simulink model "Motor_and_Driver"  (R2020a)
settings: Solver=VariableStepAuto  StartTime=0.0  StopTime=10.0  RelTol=1e-3
model workspace (MAT data in the model file):
  C = [700; 0.9999]
  K = 70.3
  KdPEPOS4 = 1
  KiIEPOS4 = 1
  KiPEPOS4 = 1
  KpIPEPOS4 = 1
  KpPEPOS4 = 1
  Ts = 0.02
  g = 0.1507
  m = 90.5176213536
  q = 0.1507
  tau = 0.0127
undefined symbols (not defined in the file): A, Angle, B, Current, DiscIntNeverNeededParam, f_DIncrEnc, Speed, Torque
libraries: fl_lib x24, nesl_utility x15, ee_lib x7, simulink x4, powerlib_meascontrol x1
settings Model: DataDictionary=MotorInfo.sldd  OrderedModelArguments=off  Creator=khoi  LastModifiedBy=khoi
settings SolverCC: AlgebraicLoopSolver=LineSearch
settings DataIOCC: SaveFormat=Structure  SaveOutput=off
settings DebuggingCC: AlgebraicLoopMsg=none
settings ModelReferenceCC: EnableParallelModelReferenceBuilds=on
settings RTWCC: GenCodeOnly=on

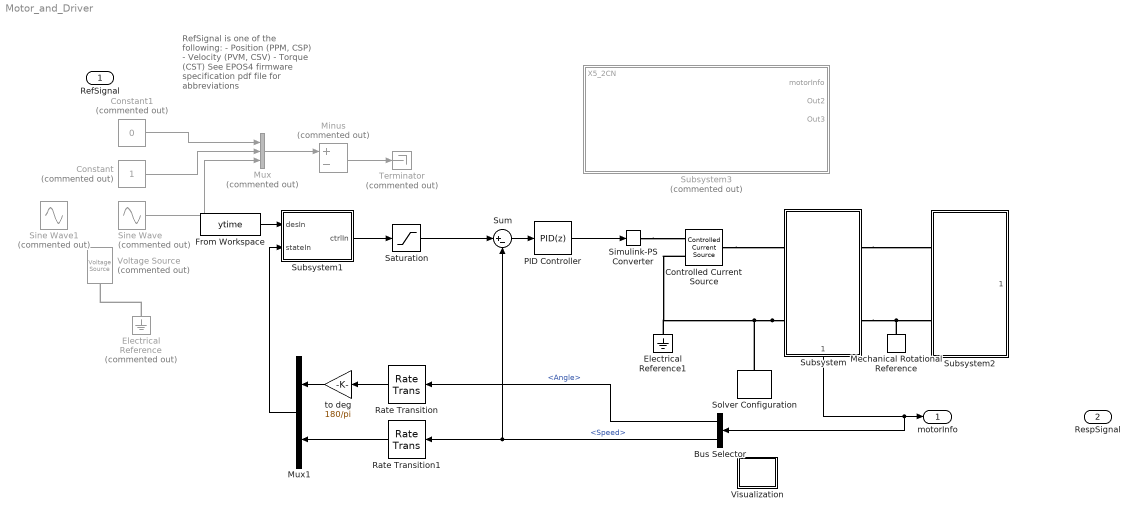
== system Motor_and_Driver ==
  note: RefSignal is one of the following:
      | - Position (PPM, CSP)
      | - Velocity (PVM, CSV)
      | - Torque (CST)
      | See EPOS4 firmware specification pdf file for abbreviations
  RefSignal : Inport
  Bus Selector : BusSelector  OutputSignals=Angle,Speed
  Constant : Constant  Commented=on
  Constant1 : Constant  Commented=on  Value=0
  Controlled Current Source : fl_lib/Electrical/Electrical Sources/Controlled Current Source
  Electrical Reference : fl_lib/Electrical/Electrical Elements/Electrical Reference  Commented=on
      settings: SourceProductBaseCode=MT,SS
  Electrical Reference1 : fl_lib/Electrical/Electrical Elements/Electrical Reference
      settings: SourceProductBaseCode=MT,SS
  From Workspace : FromWorkspace  VariableName=ytime  SampleTime=Ts  OutputAfterFinalValue=Holding final value
  Mechanical Rotational Reference : fl_lib/Mechanical/Rotational Elements/Mechanical Rotational Reference
  Minus : Sum  Commented=on  Inputs=+-
  Mux : Mux  Commented=on  Inputs=3
  Mux1 : Mux  Inputs=2
  PID Controller : simulink/Continuous/PID Controller  Controller=PID  Form=Parallel  TimeDomain=Discrete-time  UseExternalTs=off  SampleTime=Ts  IntegratorMethod=Forward Euler  FilterMethod=Forward Euler  ControllerParametersSource=internal  P=-3.52033117976818  I=-1.96454147896898  D=-0.000784751618376711  UseFilter=on  N=70.0522807561808  TunerSelectOption=Transfer Function Based (PID Tuner App)  InitialConditionSource=internal  InitialConditionForIntegrator=0  InitialConditionForFilter=0  DifferentiatorICPrevScaledInput=0  ExternalReset=none  TrackingMode=off  Kt=1  LimitOutput=on  UpperSaturationLimit=15  LowerSaturationLimit=-15  LinearizeAsGain=on  AntiWindupMode=none  Kb=1  POutMin=[]  POutMax=[]  IOutMin=[]  IOutMax=[]  DOutMin=[]  DOutMax=[]  NOutMin=[]  NOutMax=[]  SumOutMin=[]  SumOutMax=[]  SaturationOutMin=[]  SaturationOutMax=[]  PParamMin=[]  PParamMax=[]  IParamMin=[]  IParamMax=[]  DParamMin=[]  DParamMax=[]  NParamMin=[]  NParamMax=[]  KbParamMin=[]  KbParamMax=[]  KtParamMin=[]  KtParamMax=[]  KbOutMin=[]  KbOutMax=[]  KtOutMin=[]  KtOutMax=[]  IntegratorOutMin=[]  IntegratorOutMax=[]  FilterOutMin=[]  FilterOutMax=[]  SumI1OutMin=[]  SumI1OutMax=[]  SumI2OutMin=[]  SumI2OutMax=[]  SumI3OutMin=[]  SumI3OutMax=[]  SumI4OutMin=[]  SumI4OutMax=[]  SumDOutMin=[]  SumDOutMax=[]  DifferentiatorOutMin=[]  DifferentiatorOutMax=[]  FilterDiffOutCoefMin=[]  FilterDiffOutCoefMax=[]  ReciprocalOutMin=[]  ReciprocalOutMax=[]  SumDenOutMin=[]  SumDenOutMax=[]  SumNumOutMin=[]  SumNumOutMax=[]  DivideOutMin=[]  DivideOutMax=[]  UdiffTsProdOutMin=[]  UdiffTsProdOutMax=[]  NTsProdOutMin=[]  NTsProdOutMax=[]  UintegralTsProdOutMin=[]  UintegralTsProdOutMax=[]  UngainTsProdOutMin=[]  UngainTsProdOutMax=[]  IntegratorContinuousStateAttributes=''  IntegratorStateMustResolveToSignalObject=off  IntegratorRTWStateStorageClass=Auto  FilterContinuousStateAttributes=''  FilterStateMustResolveToSignalObject=off  FilterRTWStateStorageClass=Auto  ParallelPVariant=InternalParameters  IdealPVariant=Disabled  IVariant=InternalParameters  DVariant=InternalParameters  IntegratorVariant=Discrete  SatVariant=Enabled  AWVariant=Passthrough  PCopyVariant=Disabled  TRVariant=Disabled  FdbkBlocksVariant=Forward  IdealPFdbkVariant=Disabled  SatFdbkVariant=Disabled  DerivativeFilterVariant=ForwardEulerFilter  NVariant=InternalParameters  NCopyVariant=Disabled  FilterICVariant=InternalICsFilter  IntegratorICVariant=InternalICs  ExternalResetVariant=Disabled  TRSumVariant=Passthrough  SumFdbkVariant=Disabled  SumVariant=Sum_PID  TsampFilterVariant=InternalTs  TsampNgainVariant=Passthrough  TsampIntegralVariant=Passthrough
  Rate Transition : RateTransition  OutPortSampleTime=Ts
  Rate Transition1 : RateTransition  OutPortSampleTime=Ts
  Saturation : Saturate  UpperLimit=2100  LowerLimit=-2100
  Simulink-PS Converter : nesl_utility/Simulink-PS Converter  PhysicalDomain=network_engine_domain  SubClassName=ps_input  LeftPortType=input  RightPortType=output  PseudoPeriodic=off  Frequencies=[]  NoiseDistribution=none  NoiseParameters=[]  Unit=1  AffineConversion=off  FilteringAndDerivatives=provide  SimscapeFilterOrder=1  InputFilterTimeConstant=0.001  UdotUserProvided=0
  Sine Wave : Sin  Commented=on  Amplitude=5  SampleTime=0
  Sine Wave1 : Sin  Commented=on  Amplitude=400  Bias=0.5  SampleTime=Ts
  Solver Configuration : nesl_utility/Solver Configuration  PhysicalDomain=network_engine_domain  SubClassName=solver  LeftPortType=input  RightPortType=generic  Tones=[]  Harmonics=[]  SimulateNoise=off  Profile=off  UseLocalSampling=off  EnableSwitchedLinearOptims=on  FrequencyDomain=off  UseCCode=off  RelTol=0.001  AbsTol=1e-06  MinStep=1e-09  ToWorkspace=off  RevertToSquareIcSolve=off  NumHomotopyIterations=100  PhasorMode=off  PhasorModeNumHarmonics=1  DoDC=off  ResidualTolerance=1e-09  UseLocalSolver=off  LocalSolverChoice=NE_BACKWARD_EULER_ADVANCER  LocalSolverSampleTime=0.001  DoFixedCost=off  MaxNonlinIter=3  MaxModeIter=2  LinearAlgebra=auto  EquationFormulation=NE_TIME_EF  DelaysMemoryBudget=1024  AutomaticFiltering=on  FilteringTimeConstant=0.001  PartitionStorageMethod=AS_NEEDED  PartitionMemoryBudget=1024  PartitionMethod=ROBUST
  Subsystem : Subsystem  ReferencedSubsystem=Motor
      settings: PortSchema="{\"entries\":[{\"content\":{\"sides\":[{\"content\":{\"connectorIds\":[\"LConn2\",\"LConn1\"]},\"type\":\"ConnectorPlacement.EquallySpacedRectSide\",\"uuid\":\"2c9fa8b8-125e-4798-9362-86aeecc8fa1f\"},{\"content\":{\"connectorIds\":[\"LConn3\",\"LConn4\"],\"side\":\"RIGHT\"},\"type\":\"ConnectorPlacement.EquallySpacedRectSide\",\"uuid\":\"4f69e704-bc05-469f-ab35-d6b84ad80397\"},{\"content\":{\"connectorIds\":[],\"side\":\"TOP\"},\"type\":\"ConnectorPlacement.EquallySpacedRectSide\",\"uuid\":\"cfaf3aee-cd20-40cb-9288-e8b7cf9f1276\"},{\"content\":{\"connectorIds\":[\"Out1\"],\"side\":\"BOTTOM\"},\"type\":\"ConnectorPlacement.EquallySpacedRectSide\",\"uuid\":\"777429de-77ae-4f2a-b3d7-49600205512c\"}]},\"type\":\"ConnectorPlacement.EquallySpacedConnector\",\"uuid\":\"9e55bc0d-63a8-4cde-b859-9b2193dba80d\"}],\"packageUris\":[\"http://schema.mathworks.com/mf0/Connector/19700101\"],\"version\":\"1.0\"}"
  Subsystem1 : Subsystem
  Subsystem2 : Subsystem  ReferencedSubsystem=Loads
  Subsystem3 : Subsystem  Commented=on
  Sum : Sum  Inputs=|+-
  Terminator : Terminator  Commented=on
  Visualization : Subsystem
  Voltage Source : ee_lib/Sources/Voltage Source  Commented=on  dc_voltage=x607325_VNom V  ac_voltage=0 V  ac_shift=0 rad  ac_frequency=60 Hz  noise_mode=0  PSD=0 V^2/Hz  repeatability=1  auto_seed=396848355  user_seed=0  sample_time=1e-3 s  i_specify=off  i_priority=None  i=0 A  i_nominal_specify=off  i_nominal_unit=A  i_nominal_value=1  v_specify=off  v_priority=None  v=0 V  v_nominal_specify=off  v_nominal_unit=V  v_nominal_value=1
  to deg : Gain  Gain=180/pi
  motorInfo : Outport  OutDataTypeStr=Bus: motorInfo
  RespSignal : Outport  Port=2  OutDataTypeStr=Bus: RespSignal
  wires:
  Mux/1 -> Minus/1
  Subsystem/1 -> Bus Selector/1, motorInfo/1
  Minus/1 -> Terminator/1
  ? -> RespSignal/1
  Sine Wave/1 -> Mux/3
  Constant/1 -> Mux/2
  Constant1/1 -> Mux/1
  Saturation/1 -> Sum/1
  PID Controller/1 -> Simulink-PS Converter/1
  Bus Selector/2 -> Sum/2, Rate Transition1/1  "<Speed>"
  Sum/1 -> PID Controller/1
  From Workspace/1 -> Subsystem1/1(desIn)
  Subsystem1/1(ctrlIn) -> Saturation/1
  Bus Selector/1 -> Rate Transition/1  "<Angle>"
  Rate Transition/1 -> to deg/1
  to deg/1 -> Mux1/1
  Rate Transition1/1 -> Mux1/2
  Mux1/1 -> Subsystem1/2(stateIn)
  connections:
  Subsystem/LConn1 -- Solver Configuration/RConn1 -- Controlled Current Source/RConn2 -- Electrical Reference1/LConn1
  Controlled Current Source/LConn1 -- Subsystem/LConn2
  Electrical Reference/LConn1 -- Voltage Source/RConn1
  Simulink-PS Converter/RConn1 -- Controlled Current Source/RConn1
  Mechanical Rotational Reference/LConn1 -- Subsystem2/LConn2 -- Subsystem/LConn4
  Subsystem/LConn3 -- Subsystem2/LConn1

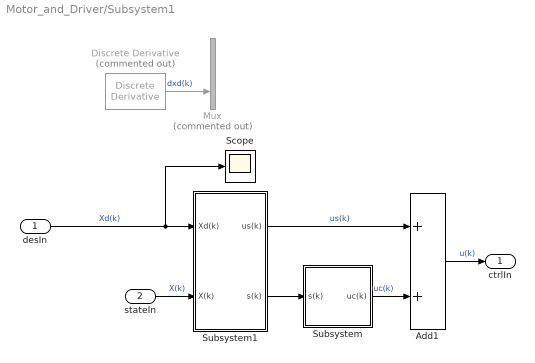
== system Motor_and_Driver/Subsystem1 ==
  desIn : Inport
  stateIn : Inport  Port=2  PortDimensions=2
  Add1 : Sum
  Discrete Derivative : simulink/Discrete/Discrete Derivative  Commented=on  gainval=1.0  ICPrevScaledInput=0.0  OutMin=[]  OutMax=[]  OutDataType=fixdt(1, 16)  OutScaling=2^-10  DoSatur=off
  Mux : Mux  Commented=on  Inputs=2
  Scope : Scope
  Subsystem : Subsystem
  Subsystem1 : Subsystem
  ctrlIn : Outport
  wires:
  desIn/1 -> Scope/1, Subsystem1/1(Xd(k))  "Xd(k)"
  Subsystem1/1(us(k)) -> Add1/1  "us(k)"
  stateIn/1 -> Subsystem1/2(X(k))  "X(k)"
  Subsystem/1(uc(k)) -> Add1/2  "uc(k)"
  Subsystem1/2(s(k)) -> Subsystem/1(s(k))
  Add1/1 -> ctrlIn/1  "u(k)"
  Discrete Derivative/1 -> Mux/2  "dxd(k)"

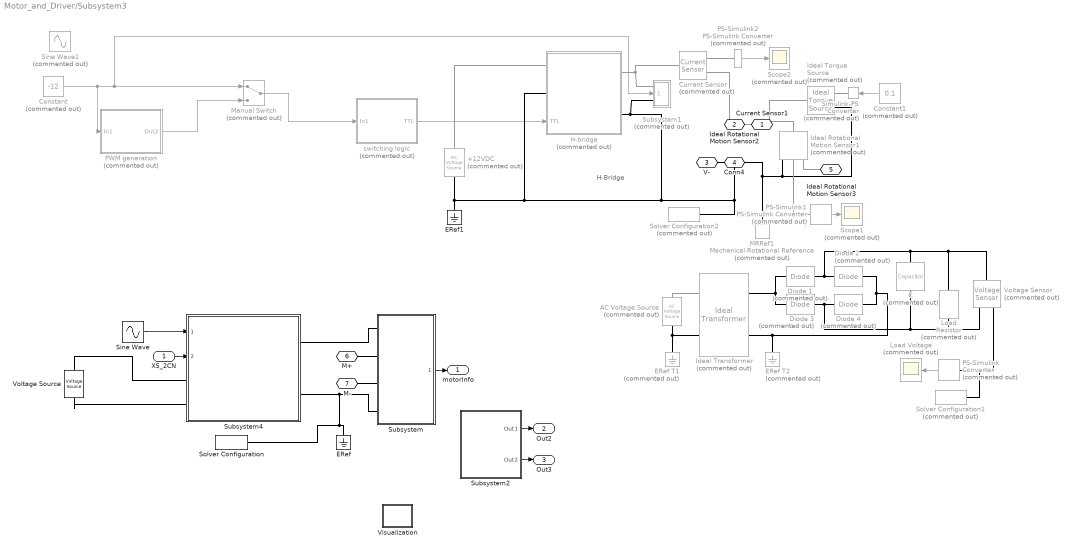
== system Motor_and_Driver/Subsystem3 ==
  note: H-Bridge
  X5_2CN : Inport
  +12VDC : fl_lib/Electrical/Electrical Sources/DC Voltage Source  Commented=on  v0=12 V
      settings: SourceProductBaseCode=MT,SS
  AC Voltage Source : fl_lib/Electrical/Electrical Sources/AC Voltage Source  Commented=on  amp=sqrt(2)*120 V  shift=0 deg  frequency=60 Hz  omega=0 rad/s
      settings: SourceProductBaseCode=MT,SS
  C : fl_lib/Electrical/Electrical Elements/Capacitor  Commented=on  c=470e-06 F  r=1e-06 Ohm  g=0 1/Ohm  i_specify=off  i_priority=High  i=0 A  i_nominal_specify=off  i_nominal_unit=A  i_nominal_value=1  v_specify=off  v_priority=High  v=0 V  v_nominal_specify=off  v_nominal_unit=V  v_nominal_value=1  vc_specify=on  vc_priority=High  vc=0 V  vc_nominal_specify=off  vc_nominal_unit=V  vc_nominal_value=1
      settings: SourceProductBaseCode=MT,SS
  Constant : Constant  Commented=on  Value=-12
  Constant1 : Constant  Commented=on  Value=0.1
  Current Sensor : fl_lib/Electrical/Electrical Sensors/Current Sensor  Commented=on
  Diode {1..4} (4 alike) : fl_lib/Electrical/Electrical Elements/Diode  Commented=on  Vf=0.6 V  Ron=0.3 Ohm  Goff=1e-08 1/Ohm  i_specify=off  i_priority=High  i=0 A  i_nominal_specify=off  i_nominal_unit=A  i_nominal_value=1  v_specify=off  v_priority=High  v=0 V  v_nominal_specify=off  v_nominal_unit=V  v_nominal_value=1
      settings: SourceProductBaseCode=MT,SS
  ERef : fl_lib/Electrical/Electrical Elements/Electrical Reference
      settings: SourceProductBaseCode=MT,SS
  ERef T1 : fl_lib/Electrical/Electrical Elements/Electrical Reference  Commented=on
      settings: SourceProductBaseCode=MT,SS
  ERef T2 : fl_lib/Electrical/Electrical Elements/Electrical Reference  Commented=on
      settings: SourceProductBaseCode=MT,SS
  ERef1 : fl_lib/Electrical/Electrical Elements/Electrical Reference
      settings: SourceProductBaseCode=MT,SS
  H-bridge : Subsystem  Commented=on
      settings: PortSchema="{\"entries\":[{\"content\":{\"sides\":[{\"content\":{\"connectorIds\":[\"LConn1\",\"LConn2\",\"In1\"]},\"type\":\"ConnectorPlacement.EquallySpacedRectSide\",\"uuid\":\"fc5f9395-6fe0-4e46-ba71-86f87805e004\"},{\"content\":{\"connectorIds\":[\"RConn1\",\"RConn2\"],\"side\":\"RIGHT\"},\"type\":\"ConnectorPlacement.EquallySpacedRectSide\",\"uuid\":\"2ca15bd9-a54f-419c-a915-39989ac75dc3\"},{\"content\":{\"connectorIds\":[],\"side\":\"TOP\"},\"type\":\"ConnectorPlacement.EquallySpacedRectSide\",\"uuid\":\"650dbc47-32e7-4b39-ba0c-96beec205e1a\"}]},\"type\":\"ConnectorPlacement.EquallySpacedConnector\",\"uuid\":\"775f97cb-687e-4894-86d4-689d0d470dfc\"}],\"packageUris\":[\"http://schema.mathworks.com/mf0/Connector/19700101\"],\"version\":\"1.0\"}"
  Ideal Rotational Motion Sensor1 : fl_lib/Mechanical/Mechanical Sensors/Ideal Rotational Motion Sensor  Commented=on  wrap_angle=simscape.enum.onoff.off  offset=0 deg
      settings: SourceProductBaseCode=MT,SS
  Ideal Torque Source : fl_lib/Mechanical/Mechanical Sources/Ideal Torque Source  Commented=on
  Ideal Transformer : fl_lib/Electrical/Electrical Elements/Ideal Transformer  Commented=on  n=14  i1_specify=off  i1_priority=High  i1=0 A  i1_nominal_specify=off  i1_nominal_unit=A  i1_nominal_value=1  v1_specify=off  v1_priority=High  v1=0 V  v1_nominal_specify=off  v1_nominal_unit=V  v1_nominal_value=1  i2_specify=off  i2_priority=High  i2=0 A  i2_nominal_specify=off  i2_nominal_unit=A  i2_nominal_value=1  v2_specify=off  v2_priority=High  v2=0 V  v2_nominal_specify=off  v2_nominal_unit=V  v2_nominal_value=1
      settings: SourceProductBaseCode=MT,SS
  Load : fl_lib/Electrical/Electrical Elements/Resistor  Commented=on  R=100 Ohm  i_specify=off  i_priority=High  i=0 A  i_nominal_specify=off  i_nominal_unit=A  i_nominal_value=1  v_specify=off  v_priority=High  v=0 V  v_nominal_specify=off  v_nominal_unit=V  v_nominal_value=1
      settings: SourceProductBaseCode=MT,SS
  Load Voltage : Scope  Commented=on
  MRRef1 : fl_lib/Mechanical/Rotational Elements/Mechanical Rotational Reference  Commented=on
      settings: SourceProductBaseCode=MT,SS
  Manual Switch : ManualSwitch  Commented=on
  PS-Simulink Converter : nesl_utility/PS-Simulink Converter  Commented=on  PhysicalDomain=network_engine_domain  SubClassName=ps_output  LeftPortType=input  RightPortType=output  PseudoPeriodic=off  Frequencies=[]  Unit=1  AffineConversion=off
      settings: SourceProductBaseCode=MT,SS
  PS-Simulink1 : nesl_utility/PS-Simulink Converter  Commented=on  PhysicalDomain=network_engine_domain  SubClassName=ps_output  LeftPortType=input  RightPortType=output  PseudoPeriodic=off  Frequencies=[]  Unit=rpm  AffineConversion=off
      settings: SourceProductBaseCode=MT,SS
  PS-Simulink2 : nesl_utility/PS-Simulink Converter  Commented=on  PhysicalDomain=network_engine_domain  SubClassName=ps_output  LeftPortType=input  RightPortType=output  PseudoPeriodic=off  Frequencies=[]  Unit=inherit  AffineConversion=off
      settings: SourceProductBaseCode=MT,SS
  PWM generation : Subsystem  Commented=on
  Scope1 : Scope  Commented=on
  Scope2 : Scope  Commented=on
  Simulink-PS Converter : nesl_utility/Simulink-PS Converter  Commented=on  PhysicalDomain=network_engine_domain  SubClassName=ps_input  LeftPortType=input  RightPortType=output  PseudoPeriodic=off  Frequencies=[]  NoiseDistribution=none  NoiseParameters=[]  Unit=1  AffineConversion=off  FilteringAndDerivatives=provide  SimscapeFilterOrder=1  InputFilterTimeConstant=0.001  UdotUserProvided=0
  Sine Wave : Sin  Amplitude=12  SampleTime=0
  Sine Wave1 : Sin  Commented=on  Amplitude=12  SampleTime=0.01
  Solver Configuration : nesl_utility/Solver Configuration  PhysicalDomain=network_engine_domain  SubClassName=solver  LeftPortType=input  RightPortType=generic  Tones=[]  Harmonics=[]  SimulateNoise=off  Profile=off  UseLocalSampling=off  EnableSwitchedLinearOptims=on  FrequencyDomain=off  UseCCode=off  RelTol=0.001  AbsTol=1e-06  MinStep=1e-09  ToWorkspace=off  RevertToSquareIcSolve=off  NumHomotopyIterations=100  PhasorMode=off  PhasorModeNumHarmonics=1  DoDC=off  ResidualTolerance=1e-9  UseLocalSolver=off  LocalSolverChoice=NE_BACKWARD_EULER_ADVANCER  LocalSolverSampleTime=5e-6  DoFixedCost=off  MaxNonlinIter=4  MaxModeIter=2  LinearAlgebra=auto  EquationFormulation=NE_TIME_EF  DelaysMemoryBudget=1024  AutomaticFiltering=on  FilteringTimeConstant=0.001  PartitionStorageMethod=AS_NEEDED  PartitionMemoryBudget=1024  PartitionMethod=FAST
      settings: SourceProductBaseCode=MT,SS
  Solver Configuration1 : nesl_utility/Solver Configuration  Commented=on  PhysicalDomain=network_engine_domain  SubClassName=solver  LeftPortType=input  RightPortType=generic  Tones=[]  Harmonics=[]  SimulateNoise=off  Profile=off  UseLocalSampling=off  EnableSwitchedLinearOptims=on  FrequencyDomain=off  UseCCode=off  RelTol=0.001  AbsTol=1e-06  MinStep=1e-09  ToWorkspace=off  RevertToSquareIcSolve=off  NumHomotopyIterations=100  PhasorMode=off  PhasorModeNumHarmonics=1  DoDC=off  ResidualTolerance=1e-9  UseLocalSolver=off  LocalSolverChoice=NE_BACKWARD_EULER_ADVANCER  LocalSolverSampleTime=.001  DoFixedCost=off  MaxNonlinIter=3  MaxModeIter=2  LinearAlgebra=auto  EquationFormulation=NE_TIME_EF  DelaysMemoryBudget=1024  AutomaticFiltering=on  FilteringTimeConstant=0.001  PartitionStorageMethod=AS_NEEDED  PartitionMemoryBudget=1024  PartitionMethod=FAST
      settings: SourceProductBaseCode=MT,SS
  Solver Configuration2 : nesl_utility/Solver Configuration  Commented=on  PhysicalDomain=network_engine_domain  SubClassName=solver  LeftPortType=input  RightPortType=generic  Tones=[]  Harmonics=[]  SimulateNoise=off  Profile=off  UseLocalSampling=off  EnableSwitchedLinearOptims=on  FrequencyDomain=off  UseCCode=off  RelTol=0.001  AbsTol=1e-06  MinStep=1e-09  ToWorkspace=off  RevertToSquareIcSolve=off  NumHomotopyIterations=100  PhasorMode=off  PhasorModeNumHarmonics=1  DoDC=off  ResidualTolerance=1e-9  UseLocalSolver=off  LocalSolverChoice=NE_BACKWARD_EULER_ADVANCER  LocalSolverSampleTime=5e-6  DoFixedCost=off  MaxNonlinIter=4  MaxModeIter=2  LinearAlgebra=auto  EquationFormulation=NE_TIME_EF  DelaysMemoryBudget=1024  AutomaticFiltering=on  FilteringTimeConstant=0.001  PartitionStorageMethod=AS_NEEDED  PartitionMemoryBudget=1024  PartitionMethod=FAST
      settings: SourceProductBaseCode=MT,SS
  Subsystem : Subsystem  ReferencedSubsystem=Motor
      settings: PortSchema="{\"entries\":[{\"content\":{\"sides\":[{\"content\":{\"connectorIds\":[\"LConn2\",\"LConn3\",\"LConn4\",\"LConn1\"]},\"type\":\"ConnectorPlacement.EquallySpacedRectSide\",\"uuid\":\"2c9fa8b8-125e-4798-9362-86aeecc8fa1f\"},{\"content\":{\"connectorIds\":[\"Out1\"],\"side\":\"RIGHT\"},\"type\":\"ConnectorPlacement.EquallySpacedRectSide\",\"uuid\":\"4f69e704-bc05-469f-ab35-d6b84ad80397\"},{\"content\":{\"connectorIds\":[],\"side\":\"TOP\"},\"type\":\"ConnectorPlacement.EquallySpacedRectSide\",\"uuid\":\"cfaf3aee-cd20-40cb-9288-e8b7cf9f1276\"}]},\"type\":\"ConnectorPlacement.EquallySpacedConnector\",\"uuid\":\"9e55bc0d-63a8-4cde-b859-9b2193dba80d\"}],\"packageUris\":[\"http://schema.mathworks.com/mf0/Connector/19700101\"],\"version\":\"1.0\"}"
  Subsystem1 : Subsystem  Commented=on
      settings: PortSchema="{\"entries\":[{\"content\":{\"sides\":[{\"content\":{\"connectorIds\":[]},\"type\":\"ConnectorPlacement.EquallySpacedRectSide\",\"uuid\":\"8985f9b9-7c8e-48a1-a039-7cc5a202e797\"},{\"content\":{\"connectorIds\":[\"RConn1\",\"In1\",\"RConn2\"],\"side\":\"RIGHT\"},\"type\":\"ConnectorPlacement.EquallySpacedRectSide\",\"uuid\":\"648da9d7-23ce-4076-bbaa-8fdefddefded\"},{\"content\":{\"connectorIds\":[],\"side\":\"TOP\"},\"type\":\"ConnectorPlacement.EquallySpacedRectSide\",\"uuid\":\"a83ba4c6-f8c4-4c80-b17f-0923e79ebda2\"}]},\"type\":\"ConnectorPlacement.EquallySpacedConnector\",\"uuid\":\"c20a9845-b952-47be-a6da-fffd20a0a984\"}],\"packageUris\":[\"http://schema.mathworks.com/mf0/Connector/19700101\"],\"version\":\"1.0\"}"
  Subsystem2 : Subsystem
  Subsystem4 : Subsystem  ReferencedSubsystem=EPOS4
      settings: PortSchema="{\"entries\":[{\"content\":{\"sides\":[{\"content\":{\"connectorIds\":[\"In1\",\"In2\",\"LConn3\",\"LConn4\"]},\"type\":\"ConnectorPlacement.EquallySpacedRectSide\",\"uuid\":\"8249666a-dc46-49ae-baa8-33cf79e5fc7b\"},{\"content\":{\"connectorIds\":[\"LConn1\",\"LConn2\"],\"side\":\"RIGHT\"},\"type\":\"ConnectorPlacement.EquallySpacedRectSide\",\"uuid\":\"4e9a76b5-906b-4ebc-b5db-652edc4ace08\"},{\"content\":{\"connectorIds\":[],\"side\":\"TOP\"},\"type\":\"ConnectorPlacement.EquallySpacedRectSide\",\"uuid\":\"b380b1e2-a062-4a47-91fb-03cda3a68908\"}]},\"type\":\"ConnectorPlacement.EquallySpacedConnector\",\"uuid\":\"57a25abc-5ab6-4e03-bd25-737af091f3a0\"}],\"packageUris\":[\"http://schema.mathworks.com/mf0/Connector/19700101\"],\"version\":\"1.0\"}"
  Visualization : Subsystem
  Voltage Sensor : fl_lib/Electrical/Electrical Sensors/Voltage Sensor  Commented=on
      settings: SourceProductBaseCode=MT,SS
  Voltage Source : ee_lib/Sources/Voltage Source  dc_voltage=18 V  ac_voltage=0 V  ac_shift=0 rad  ac_frequency=60 Hz  noise_mode=0  PSD=0 V^2/Hz  repeatability=1  auto_seed=418932850  user_seed=0  sample_time=1e-3 s  i_specify=off  i_priority=None  i=0 A  i_nominal_specify=off  i_nominal_unit=A  i_nominal_value=1  v_specify=off  v_priority=None  v=0 V  v_nominal_specify=off  v_nominal_unit=V  v_nominal_value=1
  switching logic : Subsystem  Commented=on
  Current Sensor1 : PMIOPort  Side=Right
  Ideal Rotational Motion Sensor2 : PMIOPort  Port=2  Side=Left
  V- : PMIOPort  Port=3  Side=Left
  Conn4 : PMIOPort  Port=4  Side=Left
  Ideal Rotational Motion Sensor3 : PMIOPort  Port=5  Side=Right
  M+ : PMIOPort  Port=6  Side=Left
  M- : PMIOPort  Port=7  Side=Left
  motorInfo : Outport
  Out2 : Outport  Port=2
  Out3 : Outport  Port=3
  wires:
  Constant/1 -> PWM generation/1(In1), Subsystem1/1(In1), Manual Switch/1
  switching logic/1(TTL) -> H-bridge/1(TTL)
  Constant1/1 -> Simulink-PS Converter/1
  PS-Simulink1/1 -> Scope1/1
  PS-Simulink Converter/1 -> Load Voltage/1
  Subsystem2/2(Out2) -> Out3/1
  Manual Switch/1 -> switching logic/1(In1)
  PWM generation/1(Out2) -> Manual Switch/2
  Sine Wave/1 -> Subsystem4/1
  PS-Simulink2/1 -> Scope2/1
  X5_2CN/1 -> Subsystem4/2
  Subsystem/1 -> motorInfo/1
  Subsystem2/1(Out1) -> Out2/1
  connections:
  Current Sensor/RConn2 -- Current Sensor1/RConn1
  Subsystem/LConn3 -- M+/RConn1
  Solver Configuration/RConn1 -- ERef/LConn1 -- Subsystem/LConn1 -- Subsystem4/LConn2
  H-bridge/RConn1 -- Subsystem1/RConn1 -- Current Sensor/LConn1
  Load/LConn1 -- Diode 1/RConn1 -- Diode 2/RConn1 -- C/LConn1 -- Voltage Sensor/LConn1
  Voltage Source/LConn1 -- Subsystem4/LConn3
  Simulink-PS Converter/RConn1 -- Ideal Torque Source/RConn1
  ERef1/LConn1 -- +12VDC/RConn1 -- H-bridge/LConn2 -- Subsystem1/RConn2 -- H-bridge/RConn2 -- Solver Configuration2/RConn1 -- V-/RConn1
  Load/RConn1 -- C/RConn1 -- Diode 3/LConn1 -- Diode 4/LConn1 -- Voltage Sensor/RConn2
  Voltage Source/RConn1 -- Subsystem4/LConn4
  Diode 3/RConn1 -- Ideal Transformer/RConn1 -- Diode 1/LConn1
  Diode 2/LConn1 -- Diode 4/RConn1 -- Ideal Transformer/RConn2 -- ERef T2/LConn1
  Subsystem4/LConn1 -- Subsystem/LConn2
  H-bridge/LConn1 -- +12VDC/LConn1
  MRRef1/LConn1 -- Ideal Torque Source/RConn2 -- Ideal Rotational Motion Sensor1/RConn1 -- Conn4/RConn1
  PS-Simulink Converter/LConn1 -- Voltage Sensor/RConn1 -- Solver Configuration1/RConn1
  Ideal Rotational Motion Sensor1/RConn2 -- PS-Simulink1/LConn1
  PS-Simulink2/LConn1 -- Current Sensor/RConn1
  Ideal Transformer/LConn1 -- AC Voltage Source/LConn1
  Ideal Transformer/LConn2 -- AC Voltage Source/RConn1 -- ERef T1/LConn1
  Ideal Torque Source/LConn1 -- Ideal Rotational Motion Sensor1/LConn1 -- Ideal Rotational Motion Sensor2/RConn1
  Subsystem/LConn4 -- M-/RConn1
  Ideal Rotational Motion Sensor1/RConn3 -- Ideal Rotational Motion Sensor3/RConn1

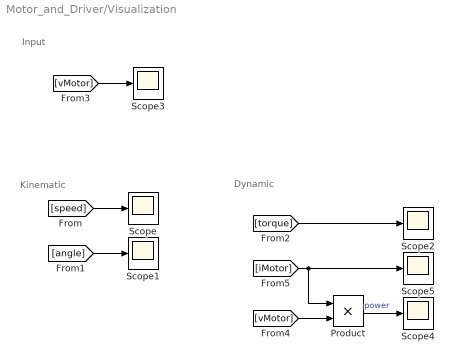
== system Motor_and_Driver/Visualization ==
  note: Dynamic
  note: Kinematic
  note: Input
  Product : Product
  Scope{,1..5} (6 alike) : Scope
  wires:
  [torque] -> Scope2/1
  [angle] -> Scope1/1
  [vMotor] -> Scope3/1
  [speed] -> Scope/1
  Product/1 -> Scope4/1  "power"
  [iMotor] -> Product/1, Scope5/1
  [vMotor] -> Product/2

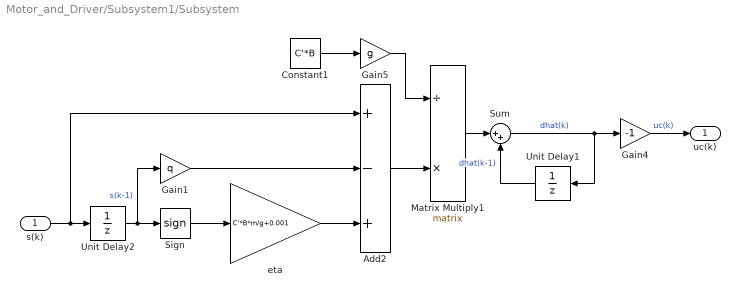
== system Motor_and_Driver/Subsystem1/Subsystem ==
  s(k) : Inport
  Add2 : Sum  Inputs=+-+
  Constant1 : Constant  Value=C'*B
  Gain1 : Gain  Gain=q
  Gain4 : Gain  Gain=-1
  Gain5 : Gain  Gain=g
  Matrix Multiply1 : Product  Inputs=/*  Multiplication=Matrix(*)
  Sign : Signum
  Sum : Sum  Inputs=|++
  Unit Delay1 : UnitDelay  SampleTime=-1  HasFrameUpgradeWarning=on
  Unit Delay2 : UnitDelay  SampleTime=-1  HasFrameUpgradeWarning=on
  eta : Gain  Gain=C'*B*m/g+0.001
  uc(k) : Outport
  wires:
  Add2/1 -> Matrix Multiply1/2
  Constant1/1 -> Gain5/1
  Gain1/1 -> Add2/2
  Gain4/1 -> uc(k)/1  "uc(k)"
  Gain5/1 -> Matrix Multiply1/1
  Unit Delay1/1 -> Sum/2  "dhat(k-1)"
  Matrix Multiply1/1 -> Sum/1
  Sum/1 -> Unit Delay1/1, Gain4/1  "dhat(k)"
  Sign/1 -> eta/1
  eta/1 -> Add2/3
  s(k)/1 -> Add2/1, Unit Delay2/1
  Unit Delay2/1 -> Sign/1, Gain1/1  "s(k-1)"

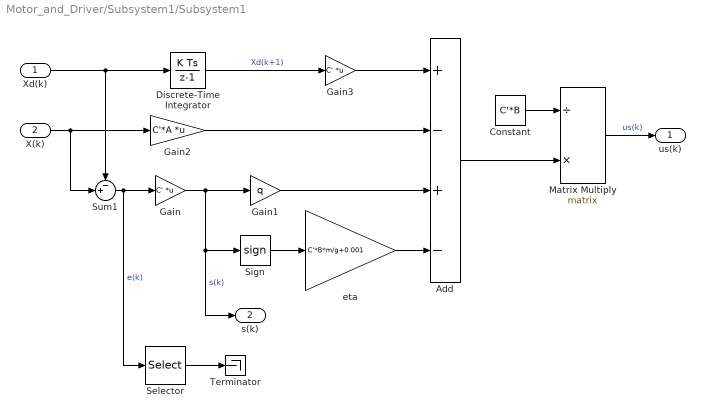
== system Motor_and_Driver/Subsystem1/Subsystem1 ==
  Xd(k) : Inport
  X(k) : Inport  Port=2
  Add : Sum  Inputs=+-+-
  Constant : Constant  Value=C'*B
  Discrete-Time Integrator : DiscreteIntegrator  SampleTime=-1  ICPrevOutput=DiscIntNeverNeededParam  ICPrevScaledInput=DiscIntNeverNeededParam
  Gain : Gain  Gain=C'  Multiplication=Matrix(K*u)
  Gain1 : Gain  Gain=q
  Gain2 : Gain  Gain=C'*A  Multiplication=Matrix(K*u)
  Gain3 : Gain  Gain=C'  Multiplication=Matrix(K*u)
  Matrix Multiply : Product  Inputs=/*  Multiplication=Matrix(*)
  Selector : Selector  InputPortWidth=2  IndexOptions=Index vector (dialog)  Indices=1  OutputSizes=1
  Sign : Signum
  Sum1 : Sum  Inputs=-+|
  Terminator : Terminator
  eta : Gain  Gain=C'*B*m/g+0.001
  us(k) : Outport
  s(k) : Outport  Port=2
  wires:
  Sign/1 -> eta/1
  Matrix Multiply/1 -> us(k)/1  "us(k)"
  eta/1 -> Add/4
  Gain2/1 -> Add/2
  Sum1/1 -> Selector/1, Gain/1  "e(k)"
  Constant/1 -> Matrix Multiply/1
  Gain1/1 -> Add/3
  Gain3/1 -> Add/1
  Add/1 -> Matrix Multiply/2
  Xd(k)/1 -> Sum1/1, Discrete-Time Integrator/1
  X(k)/1 -> Gain2/1, Sum1/2
  Gain/1 -> Sign/1, s(k)/1, Gain1/1  "s(k)"
  Discrete-Time Integrator/1 -> Gain3/1  "Xd(k+1)"
  Selector/1 -> Terminator/1

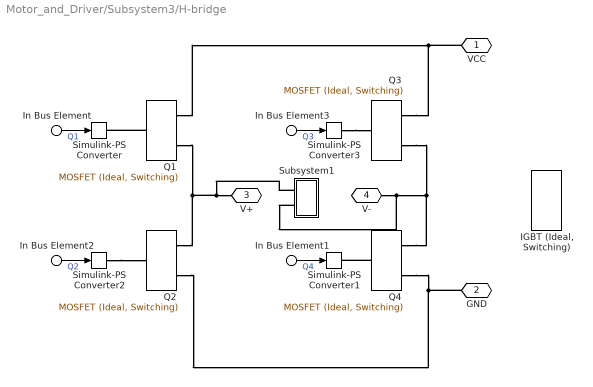
== system Motor_and_Driver/Subsystem3/H-bridge ==
  In Bus Element : Inport  PortName=TTL  Element=Forward1
  In Bus Element1 : Inport  PortName=TTL  Element=Forward2
  In Bus Element2 : Inport  PortName=TTL  Element=Reverse1
  In Bus Element3 : Inport  PortName=TTL  Element=Reverse2
  "IGBT (Ideal, Switching)" : ee_lib/Semiconductors & Converters/IGBT (Ideal, Switching)  Vf=0.8 V  Ron=0.001 Ohm  Goff=1e-5 1/Ohm  Vth=6 V  diode_param=1  diode_Vf=0.8 V  diode_Ron=0.001 Ohm  diode_Goff=1e-5 1/Ohm  diode_C=50e-9 F  diode_iRM=-235 A  diode_iF=300 A  diode_idot=-50 A/us  diode_trr_param=1  diode_trr_factor=3  diode_trr=15 us  diode_Qrr=1500 s*uA  thermal_loss_option=2  Voff=300 V  Tau=1e-4 s  Tj=[298.15, 398.15] K  Iout_scalar=600 A  Eon_scalar=22.86e-3 J  Eoff_scalar=17.14e-3 J  Von_scalar=2.7 V  Iout_data=[0, 10, 50, 100, 200, 400, 600] A  Eon_data=[0, .29, 1.43, 2.86, 5.71, 13.14, 22.86; 0, .57, 2.63, 5.14, 10.29, 20.57, 30.29] * 1e-3 J  Eoff_data=[0, .21, 1.07, 2.14, 4.29, 9.86, 17.14; 0, .43, 1.97, 3.86, 7.71, 15.43, 22.71] * 1e-3 J  Von_data=[0, 1.1, 1.3, 1.45, 1.75, 2.25, 2.7; 0, 1, 1.15, 1.35, 1.7, 2.35, 3] V
  Q{1..4} (4 alike) : ee_lib/Semiconductors & Converters/MOSFET (Ideal, Switching)  Rds=0.01 Ohm  Goff=1e-6 1/Ohm  Vth=0.5 V  diode_param=2  diode_Vf=0.4 V  diode_Ron=0.001 Ohm  diode_Goff=1e-5 1/Ohm  diode_C=50e-9 F  diode_iRM=-235 A  diode_iF=300 A  diode_idot=-50 A/us  diode_trr_param=1  diode_trr_factor=3  diode_trr=15 us  diode_Qrr=1500 s*uA  thermal_loss_option=2  Voff=300 V  Tau=1e-4 s  Tj=[298.15, 398.15] K  Iout_scalar=600 A  Eon_scalar=22.86e-3 J  Eoff_scalar=17.14e-3 J  Von_scalar=2.7 V  Iout_data=[0, 10, 50, 100, 200, 400, 600] A  Eon_data=[0, .29, 1.43, 2.86, 5.71, 13.14, 22.86; 0, .57, 2.63, 5.14, 10.29, 20.57, 30.29] * 1e-3 J  Eoff_data=[0, .21, 1.07, 2.14, 4.29, 9.86, 17.14; 0, .43, 1.97, 3.86, 7.71, 15.43, 22.71] * 1e-3 J  Von_data=[0, 1.1, 1.3, 1.45, 1.75, 2.25, 2.7; 0, 1, 1.15, 1.35, 1.7, 2.35, 3] V
  Simulink-PS Converter{,1..3} (4 alike) : nesl_utility/Simulink-PS Converter  PhysicalDomain=network_engine_domain  SubClassName=ps_input  LeftPortType=input  RightPortType=output  PseudoPeriodic=off  Frequencies=[]  NoiseDistribution=none  NoiseParameters=[]  Unit=1  AffineConversion=off  FilteringAndDerivatives=provide  SimscapeFilterOrder=1  InputFilterTimeConstant=0.001  UdotUserProvided=0
  Subsystem1 : Subsystem
  VCC : PMIOPort  Side=Left
  GND : PMIOPort  Port=2  Side=Left
  V+ : PMIOPort  Port=3  Side=Right
  V- : PMIOPort  Port=4  Side=Right
  wires:
  In Bus Element/1 -> Simulink-PS Converter/1  "Q1"
  In Bus Element1/1 -> Simulink-PS Converter1/1  "Q4"
  In Bus Element3/1 -> Simulink-PS Converter3/1  "Q3"
  In Bus Element2/1 -> Simulink-PS Converter2/1  "Q2"
  connections:
  Q4/LConn1 -- Simulink-PS Converter1/RConn1
  Simulink-PS Converter3/RConn1 -- Q3/LConn1
  V+/RConn1 -- Q1/RConn2 -- Q2/RConn1 -- Subsystem1/RConn1
  Q1/LConn1 -- Simulink-PS Converter/RConn1
  GND/RConn1 -- Q4/RConn2 -- Q2/RConn2
  VCC/RConn1 -- Q3/RConn1 -- Q1/RConn1
  V-/RConn1 -- Q4/RConn1 -- Q3/RConn2 -- Subsystem1/RConn2
  Simulink-PS Converter2/RConn1 -- Q2/LConn1

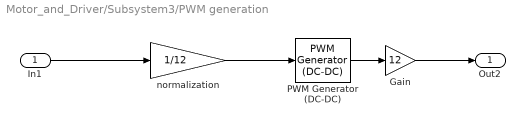
== system Motor_and_Driver/Subsystem3/PWM generation ==
  In1 : Inport
  Gain : Gain  Gain=12
  PWM Generator (DC-DC) : powerlib_meascontrol/Pulse & Signal Generators/PWM Generator (DC-DC)  Fsw=20e3  Ts=0
  normalization : Gain  Gain=1/12
  Out2 : Outport
  wires:
  PWM Generator (DC-DC)/1 -> Gain/1
  normalization/1 -> PWM Generator (DC-DC)/1
  In1/1 -> normalization/1
  Gain/1 -> Out2/1

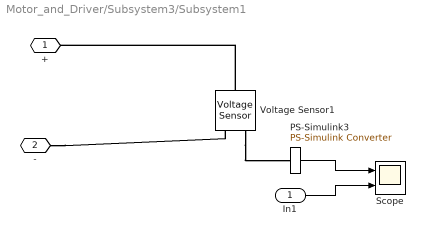
== system Motor_and_Driver/Subsystem3/Subsystem1 ==
  In1 : Inport
  PS-Simulink3 : nesl_utility/PS-Simulink Converter  PhysicalDomain=network_engine_domain  SubClassName=ps_output  LeftPortType=input  RightPortType=output  PseudoPeriodic=off  Frequencies=[]  Unit=inherit  AffineConversion=off
      settings: SourceProductBaseCode=MT,SS
  Scope : Scope  NumInputPorts=2
  Voltage Sensor1 : fl_lib/Electrical/Electrical Sensors/Voltage Sensor
  + : PMIOPort  Side=Right
  - : PMIOPort  Port=2  Side=Right
  wires:
  PS-Simulink3/1 -> Scope/1
  In1/1 -> Scope/2
  connections:
  Voltage Sensor1/RConn1 -- PS-Simulink3/LConn1
  -/RConn1 -- Voltage Sensor1/RConn2
  Voltage Sensor1/LConn1 -- +/RConn1

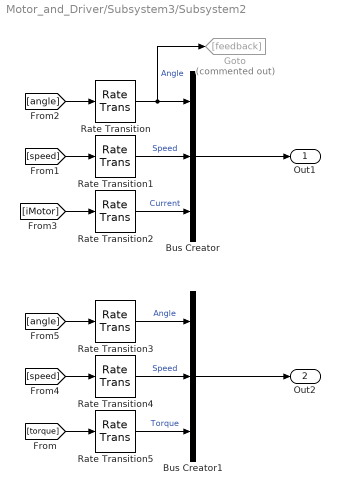
== system Motor_and_Driver/Subsystem3/Subsystem2 ==
  Bus Creator : BusCreator  Inputs=Angle,Speed,Current  OutDataTypeStr=Bus: motorInfo  NonVirtualBus=on
  Bus Creator1 : BusCreator  Inputs=Angle,Speed,Torque  OutDataTypeStr=Bus: RespSignal  NonVirtualBus=on
  Goto : Goto  Commented=on  GotoTag=feedback
  Rate Transition{,1..5} (6 alike) : RateTransition  OutPortSampleTime=1/f_DIncrEnc
  Out1 : Outport
  Out2 : Outport  Port=2
  wires:
  [iMotor] -> Rate Transition2/1
  Rate Transition5/1 -> Bus Creator1/3  "Torque"
  Rate Transition/1 -> Goto/1, Bus Creator/1  "Angle"
  [torque] -> Rate Transition5/1
  [speed] -> Rate Transition1/1
  [angle] -> Rate Transition/1
  Rate Transition2/1 -> Bus Creator/3  "Current"
  Rate Transition1/1 -> Bus Creator/2  "Speed"
  Rate Transition4/1 -> Bus Creator1/2  "Speed"
  [angle] -> Rate Transition3/1
  [speed] -> Rate Transition4/1
  Rate Transition3/1 -> Bus Creator1/1  "Angle"
  Bus Creator/1 -> Out1/1
  Bus Creator1/1 -> Out2/1

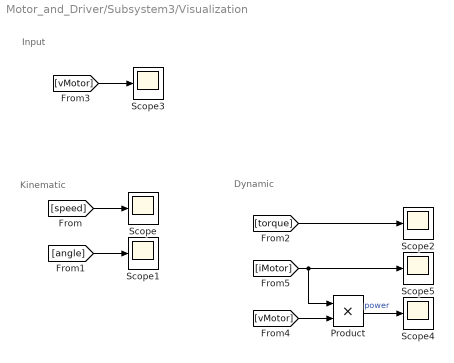
== system Motor_and_Driver/Subsystem3/Visualization ==
  note: Dynamic
  note: Kinematic
  note: Input
  Product : Product
  Scope{,1..5} (6 alike) : Scope
  wires:
  [torque] -> Scope2/1
  [angle] -> Scope1/1
  [vMotor] -> Scope3/1
  [speed] -> Scope/1
  Product/1 -> Scope4/1  "power"
  [iMotor] -> Product/1, Scope5/1
  [vMotor] -> Product/2

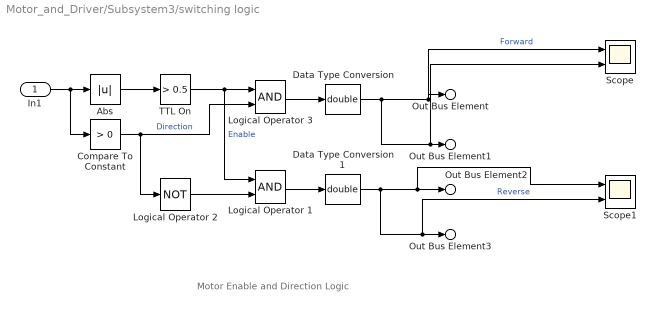
== system Motor_and_Driver/Subsystem3/switching logic ==
  note: Motor Enable and Direction Logic
  In1 : Inport
  Abs : Abs
  Compare To Constant : simulink/Logic and Bit Operations/Compare To Constant  relop=>  const=0  OutDataTypeStr=boolean  ZeroCross=off
  Data Type Conversion : DataTypeConversion  OutDataTypeStr=double
  Data Type Conversion1 : DataTypeConversion  OutDataTypeStr=double
  Logical Operator 1 : Logic  AllPortsSameDT=off  OutDataTypeStr=boolean
  Logical Operator 2 : Logic  Operator=NOT  AllPortsSameDT=off  OutDataTypeStr=boolean
  Logical Operator 3 : Logic  AllPortsSameDT=off  OutDataTypeStr=boolean
  Scope : Scope  NumInputPorts=2
  Scope1 : Scope  NumInputPorts=2
  TTL On : simulink/Logic and Bit Operations/Compare To Constant  relop=>  const=0.5  OutDataTypeStr=boolean  ZeroCross=off
  Out Bus Element : Outport  PortName=TTL  Element=Forward1
  Out Bus Element1 : Outport  PortName=TTL  Element=Forward2
  Out Bus Element2 : Outport  PortName=TTL  Element=Reverse1
  Out Bus Element3 : Outport  PortName=TTL  Element=Reverse2
  wires:
  Logical Operator 3/1 -> Data Type Conversion/1
  Logical Operator 1/1 -> Data Type Conversion1/1
  Logical Operator 2/1 -> Logical Operator 1/2
  Abs/1 -> TTL On/1
  TTL On/1 -> Logical Operator 1/1, Logical Operator 3/1  "Enable"
  In1/1 -> Abs/1, Compare To Constant/1
  Compare To Constant/1 -> Logical Operator 2/1, Logical Operator 3/2  "Direction"
  Data Type Conversion1/1 -> Scope1/1, Out Bus Element2/1, Scope1/2, Out Bus Element3/1  "Reverse"
  Data Type Conversion/1 -> Scope/1, Out Bus Element/1, Scope/2, Out Bus Element1/1  "Forward"

== system Motor_and_Driver/Subsystem3/H-bridge/Subsystem1 ==
  PS-Simulink3 : nesl_utility/PS-Simulink Converter  PhysicalDomain=network_engine_domain  SubClassName=ps_output  LeftPortType=input  RightPortType=output  PseudoPeriodic=off  Frequencies=[]  Unit=inherit  AffineConversion=off
      settings: SourceProductBaseCode=MT,SS
  Scope : Scope
  Voltage Sensor1 : fl_lib/Electrical/Electrical Sensors/Voltage Sensor
  + : PMIOPort  Side=Right
  - : PMIOPort  Port=2  Side=Right
  wires:
  PS-Simulink3/1 -> Scope/1
  connections:
  Voltage Sensor1/RConn1 -- PS-Simulink3/LConn1
  -/RConn1 -- Voltage Sensor1/RConn2
  Voltage Sensor1/LConn1 -- +/RConn1
